simulink model "PreCNN_SAC_RL_env"  (R2025b)
settings: Solver=ode4  StartTime=0.0  StopTime=50  FixedStep=0.005  RelTol=1e-3  EnableMultiTasking=on
values from neighbouring files (symbols this model uses):
  dyn_obs = struct('p0', cell(1, num_dyn_obs), 'v', cell(1, num_dyn_obs), 'radius', cell(1, num_dyn_obs))    [genera_ostacoli_dinamici.m]    (also in visualizza_raggi_completo.m = scenario.dynamic_obstacles)
  initialGainsMultiplier = 15    [init_rl.m]    (also in report_agent.m; test.m; test_agent.m; train.m)
  logging = true    [train.m]    (also in train_agent.m; train_agent_precedente.m)
  Ts = 0.1    [init_rl.m]    (also in report_agent.m; test.m; test_agent.m; train.m)
undefined symbols (not defined in the file or in its folder): angControlTuning, angRateControlTuning, bounds, Controller, decyear, DiscIntNeverNeededParam, DroneMass, Dz, Gravity, initialConditions, Iz, leapyear, logPath_num, Nz, posControlTuning, Pz, startFlightTime, tunePositionController, UAVSampleTime, Vehicle, velControlTuning
libraries: slpidlib x14, slctrl_autotuning x8, sharedutil x4, aerolibconvert2 x3, aerolibatmos2 x2, aerolibgravity2 x2, shared6dof x2, aerolibasang x2, sensorinslib x2, deeplib x1, rllib x1, matrix_library x1
(part 3 of 5)

== system PreCNN_SAC_RL_env/Inner Loop and Plant Model/High-FidelityModel/Plant Model/Bus setup/Generate GPS Data ==
  XYZ (NEU) : Inport
  "Vx, Vy, Vz" : Inport  Port=2
  DCM : Inport  Port=3
  Data Type Conversion : DataTypeConversion  OutDataTypeStr=double  SaturateOnIntegerOverflow=off  RndMeth=Floor
  Data Type Conversion1 : DataTypeConversion  OutDataTypeStr=double  SaturateOnIntegerOverflow=off  RndMeth=Floor
  GPS Model : sensorinslib/INS  Commented=through  MountingLocation=[0 0 0]  RollAccuracy=0.2  PitchAccuracy=0.2  YawAccuracy=1  PositionAccuracy=0.85  VelocityAccuracy=0.05  UseAccelAndAngVel=off  AccelerationAccuracy=0  AngularVelocityAccuracy=0  TimeInput=off  PositionErrorFactor=[0 0 0]  SeedDouble=67  SimulateUsing=Code generation
  Reshape : Reshape  OutputDimensionality=Customize  OutputDimensions=[1 3]
  Reshape1 : Reshape  OutputDimensionality=Customize  OutputDimensions=[1 3]
  "Scale and Assemble GPS Data " : Subsystem
  Terminator1 : Terminator
  Variant Source : VariantSource  VariantControlMode=label  LabelModeActiveChoice=Model  VariantControls={NoModel, Model}
  Variant Source1 : VariantSource  VariantControlMode=label  LabelModeActiveChoice=Model  VariantControls={NoModel, Model}
  GPSData : Outport  VectorParamsAs1DForOutWhenUnconnected=off
  wires:
  DCM/1 -> GPS Model/3
  "Vx, Vy, Vz"/1 -> Variant Source1/1, Reshape1/1
  XYZ (NEU)/1 -> Variant Source/1, Reshape/1
  GPS Model/3 -> Terminator1/1
  Reshape/1 -> GPS Model/1
  Reshape1/1 -> GPS Model/2
  "Scale and Assemble GPS Data "/1(Out1) -> GPSData/1
  GPS Model/1 -> Data Type Conversion1/1
  Variant Source1/1 -> "Scale and Assemble GPS Data "/2(Ve)
  GPS Model/2 -> Data Type Conversion/1
  Variant Source/1 -> "Scale and Assemble GPS Data "/1(Xe)
  Data Type Conversion/1 -> Variant Source1/2
  Data Type Conversion1/1 -> Variant Source/2

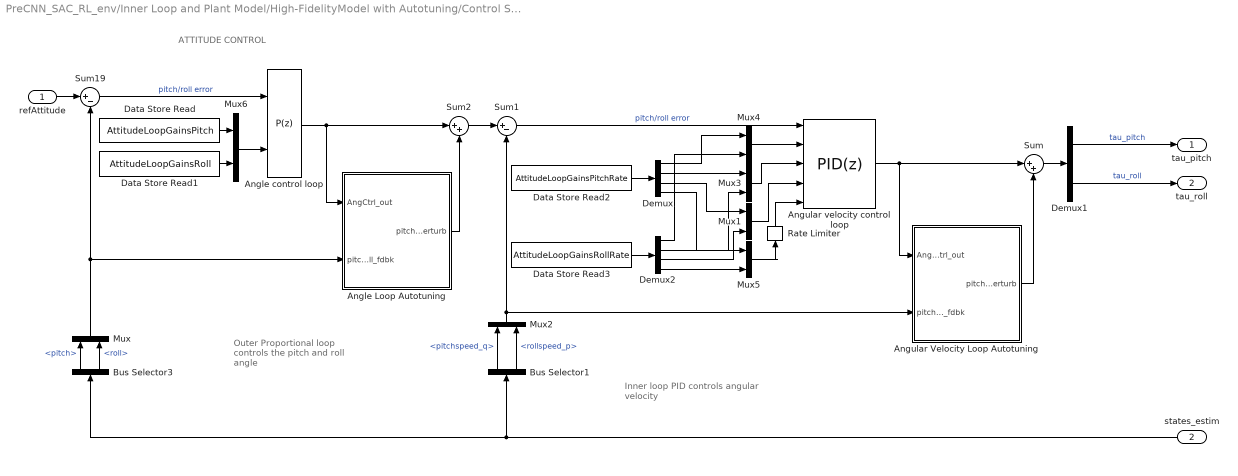
== system PreCNN_SAC_RL_env/Inner Loop and Plant Model/High-FidelityModel with Autotuning/Control System/Controller/Attitude Controller ==
  note: Inner loop PID
      | controls angular velocity
  note: Outer Proportional loop
      | controls the pitch and roll angle
  note: ATTITUDE CONTROL
  refAttitude : Inport
  states_estim : Inport  Port=2
  Angle Loop Autotuning : Subsystem
  Angle control loop : slpidlib/PID Controller  Controller=P  Form=Parallel  TimeDomain=Discrete-time  UseExternalTs=off  SampleTime=UAVSampleTime  IntegratorMethod=Forward Euler  FilterMethod=Forward Euler  ControllerParametersSource=external  P=5  I=1  UseKiTs=off  D=0  UseExternalDerivativeSource=off  N=100  UseFilter=on  TunerSelectOption=Transfer Function Based (PID Tuner App)  InitialConditionSource=internal  InitialConditionForIntegrator=0  InitialConditionForFilter=0  DifferentiatorICPrevScaledInput=0  ExternalReset=none  TrackingMode=off  Kt=1  LimitOutput=off  SatLimitsSource=internal  UpperSaturationLimit=inf  LowerSaturationLimit=-inf  LinearizeAsGain=on  AntiWindupMode=none  Kb=1  LimitIntegrator=off  UpperIntegratorSaturationLimit=inf  LowerIntegratorSaturationLimit=-inf  POutMin=[]  POutMax=[]  IOutMin=[]  IOutMax=[]  DOutMin=[]  DOutMax=[]  NOutMin=[]  NOutMax=[]  SumOutMin=[]  SumOutMax=[]  SaturationOutMin=[]  SaturationOutMax=[]  PParamMin=[]  PParamMax=[]  IParamMin=[]  IParamMax=[]  DParamMin=[]  DParamMax=[]  NParamMin=[]  NParamMax=[]  KbParamMin=[]  KbParamMax=[]  KtParamMin=[]  KtParamMax=[]  KbOutMin=[]  KbOutMax=[]  KtOutMin=[]  KtOutMax=[]  IntegratorOutMin=[]  IntegratorOutMax=[]  FilterOutMin=[]  FilterOutMax=[]  SumI1OutMin=[]  SumI1OutMax=[]  SumI2OutMin=[]  SumI2OutMax=[]  SumI3OutMin=[]  SumI3OutMax=[]  SumI4OutMin=[]  SumI4OutMax=[]  SumDOutMin=[]  SumDOutMax=[]  DifferentiatorOutMin=[]  DifferentiatorOutMax=[]  FilterDiffOutCoefMin=[]  FilterDiffOutCoefMax=[]  ReciprocalOutMin=[]  ReciprocalOutMax=[]  SumDenOutMin=[]  SumDenOutMax=[]  SumNumOutMin=[]  SumNumOutMax=[]  DivideOutMin=[]  DivideOutMax=[]  UdiffTsProdOutMin=[]  UdiffTsProdOutMax=[]  NTsProdOutMin=[]  NTsProdOutMax=[]  UintegralTsProdOutMin=[]  UintegralTsProdOutMax=[]  UngainTsProdOutMin=[]  UngainTsProdOutMax=[]  ClampingZeroOutDataTypeStr=Inherit: Inherit via back propagation  ClampingZeroOutMin=[]  ClampingZeroOutMax=[]  FilterDenConstantOutDataTypeStr=Inherit: Inherit via back propagation  FilterDenConstantOutMin=[]  FilterDenConstantOutMax=[]  PCopyOutDataTypeStr=Inherit: Inherit via back propagation  PCopyOutMin=[]  PCopyOutMax=[]  NCopyOutDataTypeStr=Inherit: Inherit via back propagation  NCopyOutMin=[]  NCopyOutMax=[]  IntegratorContinuousStateAttributes=''  IntegratorStateMustResolveToSignalObject=off  IntegratorRTWStateStorageClass=Auto  FilterContinuousStateAttributes=''  FilterStateMustResolveToSignalObject=off  FilterRTWStateStorageClass=Auto  ParallelPVariant=ExternalParameters  IdealPVariant=Disabled  IVariant=Disabled  DVariant=Disabled  IntegratorVariant=Disabled  SatVariant=Disabled  AWVariant=Disabled  PCopyVariant=Disabled  TRVariant=Disabled  FdbkBlocksVariant=Forward  IdealPFdbkVariant=Disabled  SatFdbkVariant=Disabled  DerivativeFilterVariant=Disabled  NVariant=Disabled  NCopyVariant=Disabled_SignalSpec  FilterICVariant=Disabled  IntegratorICVariant=Disabled  ExternalResetVariant=Disabled  TRSumVariant=Passthrough  SumFdbkVariant=Disabled  SumVariant=Passthrough_P  TsampFilterVariant=InternalTs  TsampNgainVariant=Passthrough  TsampIntegralVariant=Disabled_SignalSpec  ExternalSaturationOutDataTypeStr=Inherit: Same as second input  DerivativeSourceVariant=Disabled  PreIntVariant=InternalPreInt
  Angular Velocity Loop Autotuning : Subsystem
  Angular velocity control loop : slpidlib/PID Controller  Controller=PID  Form=Parallel  TimeDomain=Discrete-time  UseExternalTs=off  SampleTime=UAVSampleTime  IntegratorMethod=Forward Euler  FilterMethod=Forward Euler  ControllerParametersSource=external  P=[0.0025 .002]  I=[2*0.0025 0.003]  UseKiTs=off  D=[0.0025/25 0.003/50]  UseExternalDerivativeSource=off  N=70  UseFilter=on  TunerSelectOption=Transfer Function Based (PID Tuner App)  InitialConditionSource=internal  InitialConditionForIntegrator=0  InitialConditionForFilter=0  DifferentiatorICPrevScaledInput=0  ExternalReset=none  TrackingMode=off  Kt=1  LimitOutput=on  SatLimitsSource=internal  UpperSaturationLimit=20*pi/180  LowerSaturationLimit=-20*pi/180  LinearizeAsGain=on  AntiWindupMode=clamping  Kb=1  LimitIntegrator=off  UpperIntegratorSaturationLimit=inf  LowerIntegratorSaturationLimit=-inf  POutMin=[]  POutMax=[]  IOutMin=[]  IOutMax=[]  DOutMin=[]  DOutMax=[]  NOutMin=[]  NOutMax=[]  SumOutMin=[]  SumOutMax=[]  SaturationOutMin=[]  SaturationOutMax=[]  PParamMin=[]  PParamMax=[]  IParamMin=[]  IParamMax=[]  DParamMin=[]  DParamMax=[]  NParamMin=[]  NParamMax=[]  KbParamMin=[]  KbParamMax=[]  KtParamMin=[]  KtParamMax=[]  KbOutMin=[]  KbOutMax=[]  KtOutMin=[]  KtOutMax=[]  IntegratorOutMin=[]  IntegratorOutMax=[]  FilterOutMin=[]  FilterOutMax=[]  SumI1OutMin=[]  SumI1OutMax=[]  SumI2OutMin=[]  SumI2OutMax=[]  SumI3OutMin=[]  SumI3OutMax=[]  SumI4OutMin=[]  SumI4OutMax=[]  SumDOutMin=[]  SumDOutMax=[]  DifferentiatorOutMin=[]  DifferentiatorOutMax=[]  FilterDiffOutCoefMin=[]  FilterDiffOutCoefMax=[]  ReciprocalOutMin=[]  ReciprocalOutMax=[]  SumDenOutMin=[]  SumDenOutMax=[]  SumNumOutMin=[]  SumNumOutMax=[]  DivideOutMin=[]  DivideOutMax=[]  UdiffTsProdOutMin=[]  UdiffTsProdOutMax=[]  NTsProdOutMin=[]  NTsProdOutMax=[]  UintegralTsProdOutMin=[]  UintegralTsProdOutMax=[]  UngainTsProdOutMin=[]  UngainTsProdOutMax=[]  ClampingZeroOutDataTypeStr=Inherit: Inherit via back propagation  ClampingZeroOutMin=[]  ClampingZeroOutMax=[]  FilterDenConstantOutDataTypeStr=Inherit: Inherit via back propagation  FilterDenConstantOutMin=[]  FilterDenConstantOutMax=[]  PCopyOutDataTypeStr=Inherit: Inherit via back propagation  PCopyOutMin=[]  PCopyOutMax=[]  NCopyOutDataTypeStr=Inherit: Inherit via back propagation  NCopyOutMin=[]  NCopyOutMax=[]  IntegratorContinuousStateAttributes=''  IntegratorStateMustResolveToSignalObject=off  IntegratorRTWStateStorageClass=Auto  FilterContinuousStateAttributes=''  FilterStateMustResolveToSignalObject=off  FilterRTWStateStorageClass=Auto  ParallelPVariant=ExternalParameters  IdealPVariant=Disabled  IVariant=ExternalParameters  DVariant=ExternalParameters  IntegratorVariant=Discrete  SatVariant=Enabled  AWVariant=DiscClampingParallel  PCopyVariant=Disabled  TRVariant=Disabled  FdbkBlocksVariant=Forward  IdealPFdbkVariant=Disabled  SatFdbkVariant=Disabled  DerivativeFilterVariant=ForwardEulerFilter  NVariant=ExternalParameters  NCopyVariant=Disabled  FilterICVariant=InternalICsFilter  IntegratorICVariant=InternalICs  ExternalResetVariant=Disabled  TRSumVariant=Passthrough  SumFdbkVariant=Disabled  SumVariant=Sum_PID  TsampFilterVariant=InternalTs  TsampNgainVariant=Passthrough  TsampIntegralVariant=Disabled_SignalSpec  ExternalSaturationOutDataTypeStr=Inherit: Same as second input  DerivativeSourceVariant=ErrorSignal  PreIntVariant=InternalPreInt
  Bus Selector1 : BusSelector  OutputSignals=attitude.pitchspeed_q,attitude.rollspeed_p
  Bus Selector3 : BusSelector  OutputSignals=attitude.pitch,attitude.roll
  Data Store Read : DataStoreRead  DataStoreName=AttitudeLoopGainsPitch  IndexOptions=Index vector (dialog)  Indices=1  OutputSizes=1
  Data Store Read1 : DataStoreRead  DataStoreName=AttitudeLoopGainsRoll  IndexOptions=Index vector (dialog)  Indices=1  OutputSizes=1
  Data Store Read2 : DataStoreRead  DataStoreName=AttitudeLoopGainsPitchRate  IndexOptions=Index vector (dialog)  Indices=1  OutputSizes=1
  Data Store Read3 : DataStoreRead  DataStoreName=AttitudeLoopGainsRollRate  IndexOptions=Index vector (dialog)  Indices=1  OutputSizes=1
  Demux : Demux
  Demux1 : Demux  Outputs=2
  Demux2 : Demux
  Mux{,1..6} (7 alike) : Mux  Inputs=2
  Rate Limiter : RateLimiter  RisingSlewLimit=1000  FallingSlewLimit=-1000  SampleTimeMode=inherited
  Sum : Sum  Inputs=|++
  Sum1 : Sum  Inputs=|+-
  Sum19 : Sum  Inputs=|+-
  Sum2 : Sum  Inputs=|++
  tau_pitch : Outport  VectorParamsAs1DForOutWhenUnconnected=off
  tau_roll : Outport  Port=2  VectorParamsAs1DForOutWhenUnconnected=off
  wires:
  Sum1/1 -> Angular velocity control loop/1  "pitch/roll error"
  Mux2/1 -> Sum1/2, Angular Velocity Loop Autotuning/2(pitchrollrate_fdbk)
  Sum19/1 -> Angle control loop/1  "pitch/roll error"
  Demux1/2 -> tau_roll/1  "tau_roll"
  Demux1/1 -> tau_pitch/1  "tau_pitch"
  Bus Selector3/2 -> Mux/2  "<roll>"
  Mux/1 -> Angle Loop Autotuning/2(pitchroll_fdbk), Sum19/2
  states_estim/1 -> Bus Selector3/1, Bus Selector1/1
  Bus Selector3/1 -> Mux/1  "<pitch>"
  Bus Selector1/1 -> Mux2/1  "<pitchspeed_q>"
  Bus Selector1/2 -> Mux2/2  "<rollspeed_p>"
  Sum/1 -> Demux1/1
  Angular velocity control loop/1 -> Sum/1, Angular Velocity Loop Autotuning/1(AngVelCtrl_out)
  Angular Velocity Loop Autotuning/1(pitchrollrate_perturb) -> Sum/2
  Sum2/1 -> Sum1/1
  Angle Loop Autotuning/1(pitchroll_perturb) -> Sum2/2
  Angle control loop/1 -> Angle Loop Autotuning/1(AngCtrl_out), Sum2/1
  Data Store Read3/1 -> Demux2/1
  Data Store Read2/1 -> Demux/1
  Mux4/1 -> Angular velocity control loop/2
  Demux/1 -> Mux4/1
  Demux/2 -> Mux3/1
  Demux/3 -> Mux1/1
  Demux/4 -> Mux5/1
  Demux2/4 -> Mux5/2
  Demux2/3 -> Mux1/2
  Demux2/2 -> Mux3/2
  Demux2/1 -> Mux4/2
  Mux3/1 -> Angular velocity control loop/3
  Mux1/1 -> Angular velocity control loop/4
  Mux5/1 -> Rate Limiter/1
  refAttitude/1 -> Sum19/1
  Data Store Read1/1 -> Mux6/2
  Data Store Read/1 -> Mux6/1
  Mux6/1 -> Angle control loop/2
  Rate Limiter/1 -> Angular velocity control loop/5

== system PreCNN_SAC_RL_env/Inner Loop and Plant Model/High-FidelityModel with Autotuning/Control System/Controller/ControlMixer ==
  tau_pitch : Inport
  tau_roll : Inport  Port=2
  tau_yaw : Inport  Port=3
  totalThrust : Inport  Port=4
  Mux2 : Mux
  Product : Product  Multiplication=Matrix(*)  RndMeth=Zero
  TorqueTotalThrustToThrustPerMotor : Constant  Value=Controller.Q2Ts  OutDataTypeStr=single
  thrusts_refout : Outport  VectorParamsAs1DForOutWhenUnconnected=off
  wires:
  Product/1 -> thrusts_refout/1
  tau_roll/1 -> Mux2/4
  tau_yaw/1 -> Mux2/2
  totalThrust/1 -> Mux2/1
  TorqueTotalThrustToThrustPerMotor/1 -> Product/1
  Mux2/1 -> Product/2
  tau_pitch/1 -> Mux2/3

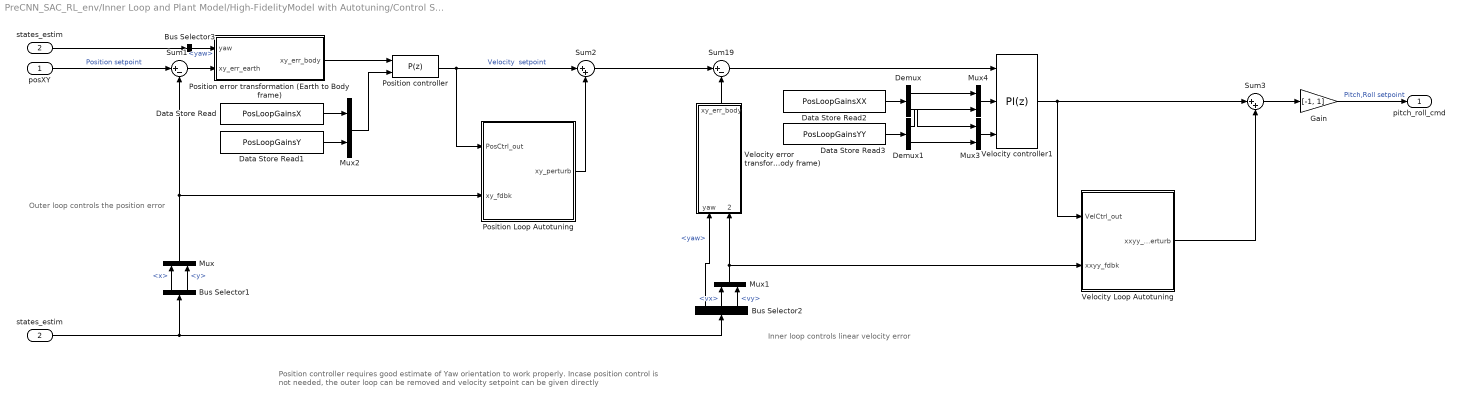
== system PreCNN_SAC_RL_env/Inner Loop and Plant Model/High-FidelityModel with Autotuning/Control System/Controller/Position Controller ==
  note: Outer loop controls the position error
  note: Inner loop controls linear velocity error
  note: Position controller requires good estimate of Yaw orientation to work properly.
      | Incase position control is not needed, the outer loop can be removed and velocity setpoint can be given directly
  posXY : Inport
  states_estim : Inport  Port=2
  Bus Selector1 : BusSelector  OutputSignals=pos_vel.x,pos_vel.y
  Bus Selector2 : BusSelector  OutputSignals=attitude.yaw,pos_vel.vx,pos_vel.vy
  Bus Selector3 : BusSelector  OutputSignals=attitude.yaw
  Data Store Read : DataStoreRead  DataStoreName=PosLoopGainsX  IndexOptions=Index vector (dialog)  Indices=1  OutputSizes=1
  Data Store Read1 : DataStoreRead  DataStoreName=PosLoopGainsY  IndexOptions=Index vector (dialog)  Indices=1  OutputSizes=1
  Data Store Read2 : DataStoreRead  DataStoreName=PosLoopGainsXX  IndexOptions=Index vector (dialog)  Indices=1  OutputSizes=1
  Data Store Read3 : DataStoreRead  DataStoreName=PosLoopGainsYY  IndexOptions=Index vector (dialog)  Indices=1  OutputSizes=1
  Demux : Demux  Outputs=2
  Demux1 : Demux  Outputs=2
  Gain : Gain  Gain=[-1, 1]
  Mux{,1..4} (5 alike) : Mux  Inputs=2
  Position Loop Autotuning : Subsystem
  Position controller : slpidlib/PID Controller  Controller=P  Form=Parallel  TimeDomain=Discrete-time  UseExternalTs=off  SampleTime=UAVSampleTime  IntegratorMethod=Forward Euler  FilterMethod=Forward Euler  ControllerParametersSource=external  P=0.25  I=0.1  UseKiTs=off  D=0  UseExternalDerivativeSource=off  N=100  UseFilter=on  TunerSelectOption=Transfer Function Based (PID Tuner App)  InitialConditionSource=internal  InitialConditionForIntegrator=0  InitialConditionForFilter=0  DifferentiatorICPrevScaledInput=0  ExternalReset=none  TrackingMode=off  Kt=1  LimitOutput=on  SatLimitsSource=internal  UpperSaturationLimit=4  LowerSaturationLimit=-4  LinearizeAsGain=on  AntiWindupMode=clamping  Kb=1  LimitIntegrator=off  UpperIntegratorSaturationLimit=inf  LowerIntegratorSaturationLimit=-inf  POutMin=[]  POutMax=[]  IOutMin=[]  IOutMax=[]  DOutMin=[]  DOutMax=[]  NOutMin=[]  NOutMax=[]  SumOutMin=[]  SumOutMax=[]  SaturationOutMin=[]  SaturationOutMax=[]  PParamMin=[]  PParamMax=[]  IParamMin=[]  IParamMax=[]  DParamMin=[]  DParamMax=[]  NParamMin=[]  NParamMax=[]  KbParamMin=[]  KbParamMax=[]  KtParamMin=[]  KtParamMax=[]  KbOutMin=[]  KbOutMax=[]  KtOutMin=[]  KtOutMax=[]  IntegratorOutMin=[]  IntegratorOutMax=[]  FilterOutMin=[]  FilterOutMax=[]  SumI1OutMin=[]  SumI1OutMax=[]  SumI2OutMin=[]  SumI2OutMax=[]  SumI3OutMin=[]  SumI3OutMax=[]  SumI4OutMin=[]  SumI4OutMax=[]  SumDOutMin=[]  SumDOutMax=[]  DifferentiatorOutMin=[]  DifferentiatorOutMax=[]  FilterDiffOutCoefMin=[]  FilterDiffOutCoefMax=[]  ReciprocalOutMin=[]  ReciprocalOutMax=[]  SumDenOutMin=[]  SumDenOutMax=[]  SumNumOutMin=[]  SumNumOutMax=[]  DivideOutMin=[]  DivideOutMax=[]  UdiffTsProdOutMin=[]  UdiffTsProdOutMax=[]  NTsProdOutMin=[]  NTsProdOutMax=[]  UintegralTsProdOutMin=[]  UintegralTsProdOutMax=[]  UngainTsProdOutMin=[]  UngainTsProdOutMax=[]  ClampingZeroOutDataTypeStr=Inherit: Inherit via back propagation  ClampingZeroOutMin=[]  ClampingZeroOutMax=[]  FilterDenConstantOutDataTypeStr=Inherit: Inherit via back propagation  FilterDenConstantOutMin=[]  FilterDenConstantOutMax=[]  PCopyOutDataTypeStr=Inherit: Inherit via back propagation  PCopyOutMin=[]  PCopyOutMax=[]  NCopyOutDataTypeStr=Inherit: Inherit via back propagation  NCopyOutMin=[]  NCopyOutMax=[]  IntegratorContinuousStateAttributes=''  IntegratorStateMustResolveToSignalObject=off  IntegratorRTWStateStorageClass=Auto  FilterContinuousStateAttributes=''  FilterStateMustResolveToSignalObject=off  FilterRTWStateStorageClass=Auto  ParallelPVariant=ExternalParameters  IdealPVariant=Disabled  IVariant=Disabled  DVariant=Disabled  IntegratorVariant=Disabled  SatVariant=Enabled  AWVariant=Disabled  PCopyVariant=Disabled  TRVariant=Disabled  FdbkBlocksVariant=Forward  IdealPFdbkVariant=Disabled  SatFdbkVariant=Disabled  DerivativeFilterVariant=Disabled  NVariant=Disabled  NCopyVariant=Disabled_SignalSpec  FilterICVariant=Disabled  IntegratorICVariant=Disabled  ExternalResetVariant=Disabled  TRSumVariant=Passthrough  SumFdbkVariant=Disabled  SumVariant=Passthrough_P  TsampFilterVariant=InternalTs  TsampNgainVariant=Passthrough  TsampIntegralVariant=Disabled_SignalSpec  ExternalSaturationOutDataTypeStr=Inherit: Same as second input  DerivativeSourceVariant=Disabled  PreIntVariant=InternalPreInt
  Position error transformation (Earth to Body frame) : MATLAB Function  TreatAsAtomicUnit=on
  Sum1 : Sum  Inputs=|+-
  Sum19 : Sum  Inputs=|+-
  Sum2 : Sum  Inputs=|++
  Sum3 : Sum  Inputs=|++
  Velocity Loop Autotuning : Subsystem
  Velocity controller1 : slpidlib/PID Controller  Controller=PI  Form=Parallel  TimeDomain=Discrete-time  UseExternalTs=off  SampleTime=UAVSampleTime  IntegratorMethod=Forward Euler  FilterMethod=Forward Euler  ControllerParametersSource=external  P=0.15  I=0.075  UseKiTs=off  D=0  UseExternalDerivativeSource=off  N=100  UseFilter=on  TunerSelectOption=Transfer Function Based (PID Tuner App)  InitialConditionSource=internal  InitialConditionForIntegrator=0  InitialConditionForFilter=0  DifferentiatorICPrevScaledInput=0  ExternalReset=none  TrackingMode=off  Kt=1  LimitOutput=on  SatLimitsSource=internal  UpperSaturationLimit=20*pi/180  LowerSaturationLimit=-20*pi/180  LinearizeAsGain=on  AntiWindupMode=clamping  Kb=1  LimitIntegrator=off  UpperIntegratorSaturationLimit=inf  LowerIntegratorSaturationLimit=-inf  POutMin=[]  POutMax=[]  IOutMin=[]  IOutMax=[]  DOutMin=[]  DOutMax=[]  NOutMin=[]  NOutMax=[]  SumOutMin=[]  SumOutMax=[]  SaturationOutMin=[]  SaturationOutMax=[]  PParamMin=[]  PParamMax=[]  IParamMin=[]  IParamMax=[]  DParamMin=[]  DParamMax=[]  NParamMin=[]  NParamMax=[]  KbParamMin=[]  KbParamMax=[]  KtParamMin=[]  KtParamMax=[]  KbOutMin=[]  KbOutMax=[]  KtOutMin=[]  KtOutMax=[]  IntegratorOutMin=[]  IntegratorOutMax=[]  FilterOutMin=[]  FilterOutMax=[]  SumI1OutMin=[]  SumI1OutMax=[]  SumI2OutMin=[]  SumI2OutMax=[]  SumI3OutMin=[]  SumI3OutMax=[]  SumI4OutMin=[]  SumI4OutMax=[]  SumDOutMin=[]  SumDOutMax=[]  DifferentiatorOutMin=[]  DifferentiatorOutMax=[]  FilterDiffOutCoefMin=[]  FilterDiffOutCoefMax=[]  ReciprocalOutMin=[]  ReciprocalOutMax=[]  SumDenOutMin=[]  SumDenOutMax=[]  SumNumOutMin=[]  SumNumOutMax=[]  DivideOutMin=[]  DivideOutMax=[]  UdiffTsProdOutMin=[]  UdiffTsProdOutMax=[]  NTsProdOutMin=[]  NTsProdOutMax=[]  UintegralTsProdOutMin=[]  UintegralTsProdOutMax=[]  UngainTsProdOutMin=[]  UngainTsProdOutMax=[]  ClampingZeroOutDataTypeStr=Inherit: Inherit via back propagation  ClampingZeroOutMin=[]  ClampingZeroOutMax=[]  FilterDenConstantOutDataTypeStr=Inherit: Inherit via back propagation  FilterDenConstantOutMin=[]  FilterDenConstantOutMax=[]  PCopyOutDataTypeStr=Inherit: Inherit via back propagation  PCopyOutMin=[]  PCopyOutMax=[]  NCopyOutDataTypeStr=Inherit: Inherit via back propagation  NCopyOutMin=[]  NCopyOutMax=[]  IntegratorContinuousStateAttributes=''  IntegratorStateMustResolveToSignalObject=off  IntegratorRTWStateStorageClass=Auto  FilterContinuousStateAttributes=''  FilterStateMustResolveToSignalObject=off  FilterRTWStateStorageClass=Auto  ParallelPVariant=ExternalParameters  IdealPVariant=Disabled  IVariant=ExternalParameters  DVariant=Disabled  IntegratorVariant=Discrete  SatVariant=Enabled  AWVariant=DiscClampingParallel  PCopyVariant=Disabled  TRVariant=Disabled  FdbkBlocksVariant=Forward  IdealPFdbkVariant=Disabled  SatFdbkVariant=Disabled  DerivativeFilterVariant=Disabled  NVariant=Disabled  NCopyVariant=Disabled_SignalSpec  FilterICVariant=Disabled  IntegratorICVariant=InternalICs  ExternalResetVariant=Disabled  TRSumVariant=Passthrough  SumFdbkVariant=Disabled  SumVariant=Sum_PI  TsampFilterVariant=InternalTs  TsampNgainVariant=Passthrough  TsampIntegralVariant=Disabled_SignalSpec  ExternalSaturationOutDataTypeStr=Inherit: Same as second input  DerivativeSourceVariant=Disabled  PreIntVariant=InternalPreInt
  Velocity error transformation (Earth to Body frame) : MATLAB Function  TreatAsAtomicUnit=on
  "states_estim " : InportShadow  Port=2
  pitch_roll_cmd : Outport  VectorParamsAs1DForOutWhenUnconnected=off
  wires:
  Mux1/1 -> Velocity error transformation (Earth to Body frame)/2(xy_err_earth), Velocity Loop Autotuning/2(xxyy_fdbk)
  Bus Selector3/1 -> Position error transformation (Earth to Body frame)/1(yaw)  "<yaw>"
  posXY/1 -> Sum1/1  "Position setpoint"
  Position error transformation (Earth to Body frame)/1(xy_err_body) -> Position controller/1
  Mux/1 -> Sum1/2, Position Loop Autotuning/2(xy_fdbk)
  Position controller/1 -> Position Loop Autotuning/1(PosCtrl_out), Sum2/1  "Velocity  setpoint"
  Velocity controller1/1 -> Velocity Loop Autotuning/1(VelCtrl_out), Sum3/1
  Gain/1 -> pitch_roll_cmd/1  "Pitch,Roll setpoint"
  Sum19/1 -> Velocity controller1/1
  Bus Selector2/3 -> Mux1/2  "<vy>"
  Bus Selector1/2 -> Mux/2  "<y>"
  Bus Selector1/1 -> Mux/1  "<x>"
  states_estim/1 -> Bus Selector2/1, Bus Selector1/1
  Bus Selector2/2 -> Mux1/1  "<vx>"
  Bus Selector2/1 -> Velocity error transformation (Earth to Body frame)/1(yaw)  "<yaw>"
  "states_estim "/1 -> Bus Selector3/1
  Velocity error transformation (Earth to Body frame)/1(xy_err_body) -> Sum19/2
  Sum2/1 -> Sum19/1
  Position Loop Autotuning/1(xy_perturb) -> Sum2/2
  Sum3/1 -> Gain/1
  Velocity Loop Autotuning/1(xxyy_perturb) -> Sum3/2
  Sum1/1 -> Position error transformation (Earth to Body frame)/2(xy_err_earth)
  Data Store Read/1 -> Mux2/1
  Data Store Read1/1 -> Mux2/2
  Mux2/1 -> Position controller/2
  Data Store Read2/1 -> Demux/1
  Mux4/1 -> Velocity controller1/2
  Mux3/1 -> Velocity controller1/3
  Demux/1 -> Mux4/1
  Demux/2 -> Mux3/1
  Data Store Read3/1 -> Demux1/1
  Demux1/1 -> Mux4/2
  Demux1/2 -> Mux3/2

== system PreCNN_SAC_RL_env/Inner Loop and Plant Model/High-FidelityModel with Autotuning/Control System/Controller/Yaw Controller ==
  note: Yaw estimation is done solely using the gyroscope and it may drift with time.
  yaw_ref : Inport
  states_estim : Inport  Port=2
  Bus Selector1 : BusSelector  OutputSignals=attitude.yawspeed_r
  Bus Selector5 : BusSelector  OutputSignals=attitude.yaw
  D_yaw : Gain  Gain=.0006
  Discrete-Time Integrator : DiscreteIntegrator  gainval=1  SampleTime=-1  LimitOutput=on  UpperSaturationLimit=0.25  LowerSaturationLimit=-0.25  ICPrevOutput=DiscIntNeverNeededParam  ICPrevScaledInput=DiscIntNeverNeededParam
  I_yaw : Gain  Gain=0.002  ParamDataTypeStr=single  OutDataTypeStr=single
  MATLAB Function : MATLAB Function  TreatAsAtomicUnit=on
  MATLAB Function1 : MATLAB Function  TreatAsAtomicUnit=on
  P_yaw : Gain  Gain=0.006  ParamDataTypeStr=single  OutDataTypeStr=single
  Sum1 : Sum  Inputs=|+-  OutDataTypeStr=single  AccumDataTypeStr=single  SaturateOnIntegerOverflow=on
  Sum2 : Sum  Inputs=++-
  tau_yaw : Outport  VectorParamsAs1DForOutWhenUnconnected=off
  wires:
  MATLAB Function1/1(y) -> P_yaw/1, I_yaw/1
  MATLAB Function/1(y) -> Sum1/1
  Discrete-Time Integrator/1 -> Sum2/2
  yaw_ref/1 -> MATLAB Function/1(u)
  Sum1/1 -> MATLAB Function1/1(u)
  D_yaw/1 -> Sum2/3
  P_yaw/1 -> Sum2/1
  Bus Selector1/1 -> D_yaw/1  "<yawspeed_r>"
  states_estim/1 -> Bus Selector5/1, Bus Selector1/1
  Bus Selector5/1 -> Sum1/2  "<yaw>"
  Sum2/1 -> tau_yaw/1
  I_yaw/1 -> Discrete-Time Integrator/1

== system PreCNN_SAC_RL_env/Inner Loop and Plant Model/High-FidelityModel with Autotuning/Control System/Controller/gravity feedforward//equilibrium thrust ==
  note: ALTITUDE
  states_estim : Inport
  PosZ : Inport  Port=2
  Bus Selector1 : BusSelector  OutputSignals=pos_vel.z,pos_vel.vz
  D_z1 : Gain  Gain=0.75  ParamDataTypeStr=single  OutDataTypeStr=single  SaturateOnIntegerOverflow=on
  Discrete-Time Integrator : DiscreteIntegrator  SampleTime=UAVSampleTime  LimitOutput=on  UpperSaturationLimit=2  LowerSaturationLimit=-2  ICPrevOutput=DiscIntNeverNeededParam  ICPrevScaledInput=DiscIntNeverNeededParam
  I_pr : Gain  Gain=0.075
  P_z1 : Gain  Gain=0.65  ParamDataTypeStr=single  OutDataTypeStr=single  SaturateOnIntegerOverflow=on
  SaturationThrust1 : Saturate  UpperLimit=4*Controller.totalThrustMaxRelative*Controller.motorsThrustPerMotorMax  LowerLimit=-4*Controller.totalThrustMaxRelative*Controller.motorsThrustPerMotorMax  OutDataTypeStr=single
  Sum1 : Sum  Inputs=++-  OutDataTypeStr=single  AccumDataTypeStr=single  SaturateOnIntegerOverflow=on
  Sum2 : Sum  Inputs=+-|  OutDataTypeStr=single  AccumDataTypeStr=single  SaturateOnIntegerOverflow=on
  Sum5 : Sum  Inputs=++|  OutDataTypeStr=single  AccumDataTypeStr=single  SaturateOnIntegerOverflow=on
  w1 : Constant  Value=-Gravity*Vehicle.Airframe.mass  OutDataTypeStr=single
  altitude_cmd : Outport  VectorParamsAs1DForOutWhenUnconnected=off
  wires:
  I_pr/1 -> Discrete-Time Integrator/1
  Sum5/1 -> SaturationThrust1/1
  Discrete-Time Integrator/1 -> Sum1/1
  D_z1/1 -> Sum1/3  "dz"
  Sum2/1 -> I_pr/1, P_z1/1  "pitch/roll error"
  Bus Selector1/2 -> D_z1/1  "<vz>"
  P_z1/1 -> Sum1/2
  states_estim/1 -> Bus Selector1/1
  Bus Selector1/1 -> Sum2/2  "<z>"
  PosZ/1 -> Sum2/1
  Sum1/1 -> Sum5/2
  SaturationThrust1/1 -> altitude_cmd/1
  w1/1 -> Sum5/1

== system PreCNN_SAC_RL_env/Inner Loop and Plant Model/High-FidelityModel with Autotuning/Control System/Controller/thrustsToMotorCommands ==
  thrusts_refin : Inport
  MotorDirections : Gain  Gain=[1 -1 1 -1]
  Saturation5 : Saturate  UpperLimit=Vehicle.Motor.maxLimit  LowerLimit=Vehicle.Motor.minLimit
  ThrustToMotorCommand : Gain  Gain=-Vehicle.Motor.thrustToMotorCommand
  motors_cmdout : Outport  VectorParamsAs1DForOutWhenUnconnected=off
  wires:
  Saturation5/1 -> MotorDirections/1
  MotorDirections/1 -> motors_cmdout/1
  ThrustToMotorCommand/1 -> Saturation5/1
  thrusts_refin/1 -> ThrustToMotorCommand/1

== system PreCNN_SAC_RL_env/Inner Loop and Plant Model/High-FidelityModel with Autotuning/Plant Model/AC model/Applied Force Calculation ==
  gravity force : Inport  Unit=N
  Aerodynamic Forces : Inport  Port=2  Unit=N
  Motor Forces : Inport  Port=3  Unit=N
  Add1 : Sum  Inputs=+++
  Signal Specification : SignalSpecification  Dimensions=3
  External Forces : Outport  Unit=N  VectorParamsAs1DForOutWhenUnconnected=off
  wires:
  Add1/1 -> Signal Specification/1
  Motor Forces/1 -> Add1/3  "Motor Thrust"
  Aerodynamic Forces/1 -> Add1/2
  gravity force/1 -> Add1/1
  Signal Specification/1 -> External Forces/1

== system PreCNN_SAC_RL_env/Inner Loop and Plant Model/High-FidelityModel with Autotuning/Plant Model/AC model/Drag Calculation ==
  Density : Inport  Unit=kg/m^3
  Vb : Inport  Port=2  Unit=m/second
  Drag Calc : Subsystem
  Gain3 : Gain  Gain=-1
  Product : Product  RndMeth=Zero
  Sign : Signum  ZeroCross=off
  Drag : Outport  Unit=N  VectorParamsAs1DForOutWhenUnconnected=off
  wires:
  Density/1 -> Drag Calc/1(Density)
  Sign/1 -> Gain3/1
  Drag Calc/1(drag) -> Product/1
  Gain3/1 -> Product/2
  Product/1 -> Drag/1  "xDrag"
  Vb/1 -> Sign/1, Drag Calc/2(vel)

== system PreCNN_SAC_RL_env/Inner Loop and Plant Model/High-FidelityModel with Autotuning/Plant Model/AC model/Gravity Force Calculation ==
  DCMbe : Inport
  gravity : Inport  Port=2  Unit=m/s^2
  Gain1 : Gain  Gain=Vehicle.Airframe.mass
  Product : Product  Multiplication=Matrix(*)
  gravity force : Outport  Unit=N  VectorParamsAs1DForOutWhenUnconnected=off
  wires:
  gravity/1 -> Gain1/1
  Gain1/1 -> Product/2  "gravity force NED"
  Product/1 -> gravity force/1
  DCMbe/1 -> Product/1

== system PreCNN_SAC_RL_env/Inner Loop and Plant Model/High-FidelityModel with Autotuning/Plant Model/AC model/Motor Forces and Torques ==
  Vb : Inport
  Density : Inport  Port=2
  pqr : Inport  Port=3
  Motor Commands : Inport  Port=4
  D1 : Constant  Value=[Vehicle.Airframe.xy -Vehicle.Airframe.xy Vehicle.Airframe.h]
  D2 : Constant  Value=[Vehicle.Airframe.xy Vehicle.Airframe.xy Vehicle.Airframe.h]
  D3 : Constant  Value=[-Vehicle.Airframe.xy Vehicle.Airframe.xy Vehicle.Airframe.h]
  D4 : Constant  Value=[-Vehicle.Airframe.xy -Vehicle.Airframe.xy Vehicle.Airframe.h]
  For Each Subsystem : Subsystem  TreatAsAtomicUnit=on
  MotorsToW : Subsystem
  Sum of Elements : Sum  Inputs=+  CollapseMode=Specified dimension  CollapseDim=2
  Sum of Elements1 : Sum  Inputs=+  CollapseMode=Specified dimension  CollapseDim=2
  Vector Concatenate : Concatenate  NumInputs=4  Mode=Multidimensional array  ConcatenateDimension=2
  Motor Forces : Outport  Unit=N  VectorParamsAs1DForOutWhenUnconnected=off
  Motor Torques : Outport  Port=2  Unit=N*m  VectorParamsAs1DForOutWhenUnconnected=off
  wires:
  D4/1 -> Vector Concatenate/4
  MotorsToW/1(omegas_datout) -> For Each Subsystem/4(w)
  Vector Concatenate/1 -> For Each Subsystem/5(D)
  For Each Subsystem/2(Moments) -> Sum of Elements1/1
  pqr/1 -> For Each Subsystem/3(Omega)
  Vb/1 -> For Each Subsystem/1(Vb)
  Motor Commands/1 -> MotorsToW/1(motors_datin)
  D1/1 -> Vector Concatenate/1
  D3/1 -> Vector Concatenate/3
  D2/1 -> Vector Concatenate/2
  Sum of Elements1/1 -> Motor Torques/1
  Density/1 -> For Each Subsystem/2(rho)
  Sum of Elements/1 -> Motor Forces/1
  For Each Subsystem/1(Forces) -> Sum of Elements/1

== system PreCNN_SAC_RL_env/Inner Loop and Plant Model/High-FidelityModel with Autotuning/Plant Model/Bus setup/Generate GPS Data ==
  XYZ (NEU) : Inport
  "Vx, Vy, Vz" : Inport  Port=2
  DCM : Inport  Port=3
  GPS Model : sensorinslib/INS  MountingLocation=[0 0 0]  RollAccuracy=0.2  PitchAccuracy=0.2  YawAccuracy=1  PositionAccuracy=0.85  VelocityAccuracy=0.05  UseAccelAndAngVel=off  AccelerationAccuracy=0  AngularVelocityAccuracy=0  TimeInput=off  PositionErrorFactor=[0 0 0]  SeedDouble=67  SimulateUsing=Code generation
  Reshape : Reshape  OutputDimensionality=Customize  OutputDimensions=[1 3]
  Reshape1 : Reshape  OutputDimensionality=Customize  OutputDimensions=[1 3]
  "Scale and Assemble GPS Data " : Subsystem
  Terminator1 : Terminator
  Variant Source : VariantSource  VariantControlMode=label  LabelModeActiveChoice=Model  VariantControls={NoModel, Model}
  Variant Source1 : VariantSource  VariantControlMode=label  LabelModeActiveChoice=Model  VariantControls={NoModel, Model}
  GPSData : Outport  VectorParamsAs1DForOutWhenUnconnected=off
  wires:
  DCM/1 -> GPS Model/3
  "Vx, Vy, Vz"/1 -> Variant Source1/1, Reshape1/1
  XYZ (NEU)/1 -> Variant Source/1, Reshape/1
  GPS Model/3 -> Terminator1/1
  Reshape/1 -> GPS Model/1
  Reshape1/1 -> GPS Model/2
  "Scale and Assemble GPS Data "/1(Out1) -> GPSData/1
  GPS Model/1 -> Variant Source/2
  Variant Source1/1 -> "Scale and Assemble GPS Data "/2(Ve)
  GPS Model/2 -> Variant Source1/2
  Variant Source/1 -> "Scale and Assemble GPS Data "/1(Xe)

== system PreCNN_SAC_RL_env/Inner Loop and Plant Model/High-FidelityModel/Plant Model/AC model/Drag Calculation/Drag Calc ==
  Density : Inport  Unit=kg/m^3
  vel : Inport  Port=2  Unit=m/s
  Dynamic Pressure : aerolibasang/Dynamic Pressure
  Gain : Gain  Gain=[.25 .25]
  Mux1 : Mux  Inputs=2
  Product : Product  Inputs=3  RndMeth=Zero
  diameter : Constant  Value=Vehicle.Airframe.diameter  SampleTime=0
  dragCoeff : Constant  Value=Vehicle.Airframe.Cdx  SampleTime=0
  drag : Outport  Unit=N  VectorParamsAs1DForOutWhenUnconnected=off
  wires:
  Product/1 -> drag/1
  dragCoeff/1 -> Product/3  "Cd"
  Dynamic Pressure/1 -> Product/1  "q"
  diameter/1 -> Gain/1, Mux1/2
  Mux1/1 -> Product/2  "S"
  Gain/1 -> Mux1/1
  vel/1 -> Dynamic Pressure/1
  Density/1 -> Dynamic Pressure/2

== system PreCNN_SAC_RL_env/Inner Loop and Plant Model/High-FidelityModel/Plant Model/AC model/Motor Forces and Torques/For Each Subsystem ==
  Vb : Inport  PortDimensions=3
  rho : Inport  Port=2  PortDimensions=1
  Omega : Inport  Port=3
  w : Inport  Port=4  Partition=on  PartitionDimension=2  PartitionWidth=1  PartitionOffset=0
  D : Inport  Port=5  Partition=on  PartitionDimension=2  PartitionWidth=1  PartitionOffset=0
  For Each : ForEach  DisableCoverage=on
  RotorDynamics : Subsystem  TreatAsAtomicUnit=on
      mask init:
      | aeroicon('aeroblk');
      settings: RTWFcnNameOpts=Use subsystem name  RTWFileNameOpts=Use function name
  Forces : Outport  ConcatenationDimension=2  VectorParamsAs1DForOutWhenUnconnected=off
  Moments : Outport  Port=2  ConcatenationDimension=2  VectorParamsAs1DForOutWhenUnconnected=off
  wires:
  RotorDynamics/1(Fxyz) -> Forces/1
  RotorDynamics/2(Mxyz) -> Moments/1
  Vb/1 -> RotorDynamics/1(Vb)
  Omega/1 -> RotorDynamics/2(pqr)
  rho/1 -> RotorDynamics/3(rho)
  D/1 -> RotorDynamics/5(Arm)
  w/1 -> RotorDynamics/4(w)

== system PreCNN_SAC_RL_env/Inner Loop and Plant Model/High-FidelityModel/Plant Model/AC model/Motor Forces and Torques/MotorsToW ==
  motors_datin : Inport
  Motordirections : Gain  Gain=[1 -1 1 -1]  ParamDataTypeStr=single  OutDataTypeStr=Inherit: Inherit via back propagation  SaturateOnIntegerOverflow=on
  Motordirections1 : Gain  Gain=[1 -1 1 -1]  ParamDataTypeStr=single  OutDataTypeStr=Inherit: Inherit via back propagation  SaturateOnIntegerOverflow=on
  Saturation5 : Saturate  UpperLimit=Vehicle.Motor.maxLimit  LowerLimit=Vehicle.Motor.minLimit  OutDataTypeStr=Inherit: Inherit via back propagation
  Signed Sqrt : Sqrt  Operator=signedSqrt  OutDataTypeStr=Inherit: Inherit via back propagation
  motorsToW2_Gain : Gain  Gain=Vehicle.Motor.commandToW2Gain  ParamDataTypeStr=single  OutDataTypeStr=Inherit: Inherit via back propagation  SaturateOnIntegerOverflow=on
  omegas_datout : Outport  VectorParamsAs1DForOutWhenUnconnected=off
  wires:
  motorsToW2_Gain/1 -> Signed Sqrt/1
  Motordirections/1 -> Saturation5/1
  Saturation5/1 -> Motordirections1/1
  Motordirections1/1 -> motorsToW2_Gain/1
  Signed Sqrt/1 -> omegas_datout/1
  motors_datin/1 -> Motordirections/1

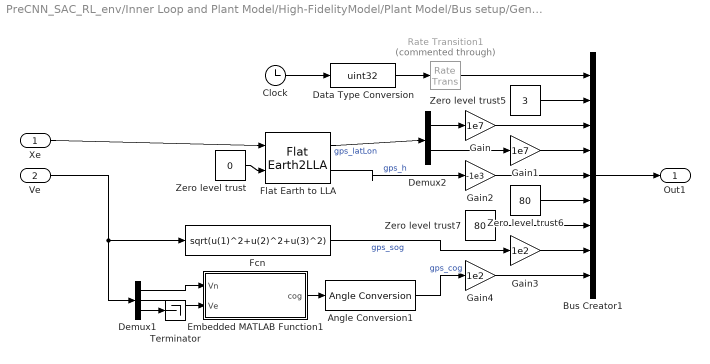
== system PreCNN_SAC_RL_env/Inner Loop and Plant Model/High-FidelityModel/Plant Model/Bus setup/Generate GPS Data/Scale and Assemble GPS Data  ==
  Xe : Inport
  Ve : Inport  Port=2
  Angle Conversion1 : aerolibconvert2/Angle Conversion  IU=rad  OU=deg
  Bus Creator1 : BusCreator  Inputs=9  OutDataTypeStr=Bus: gps_raw_int  NonVirtualBus=on
      settings: InheritFromInputs=off
  Clock : Clock
      settings: AttributesFormatString=Decimation: %<Decimation>
  Data Type Conversion : DataTypeConversion  OutDataTypeStr=uint32  SaturateOnIntegerOverflow=off  RndMeth=Floor
  Demux1 : Demux  Outputs=3
  Demux2 : Demux  Outputs=2
  Embedded MATLAB Function1 : MATLAB Function  TreatAsAtomicUnit=on
  Fcn : Fcn  Expr=sqrt(u(1)^2+u(2)^2+u(3)^2)
  Flat Earth to LLA : FlatEarth2LLA  R=6378137  LL0=uavIC_latLon
  Gain : Gain  Gain=1e7  OutDataTypeStr=int32
  Gain1 : Gain  Gain=1e7  OutDataTypeStr=int32
  Gain2 : Gain  Gain=-1e3  OutDataTypeStr=int32
  Gain3 : Gain  Gain=1e2  OutDataTypeStr=uint16
  Gain4 : Gain  Gain=1e2  OutDataTypeStr=uint16
  Rate Transition1 : RateTransition  Commented=through  OutPortSampleTime=0.005
  Terminator : Terminator
  Zero level trust : Constant  Value=0
      settings: AttributesFormatString=%<Value>
  Zero level trust5 : Constant  Value=3  OutDataTypeStr=uint8
      settings: AttributesFormatString=%<Value>
  Zero level trust6 : Constant  Value=80  OutDataTypeStr=uint16
      settings: AttributesFormatString=%<Value>
  Zero level trust7 : Constant  Value=80  OutDataTypeStr=uint16
      settings: AttributesFormatString=%<Value>
  Out1 : Outport
  wires:
  Demux2/1 -> Gain/1
  Gain/1 -> Bus Creator1/3
  Gain4/1 -> Bus Creator1/9
  Demux2/2 -> Gain1/1
  Embedded MATLAB Function1/1(cog) -> Angle Conversion1/1
  Rate Transition1/1 -> Bus Creator1/1
  Zero level trust6/1 -> Bus Creator1/6
  Gain3/1 -> Bus Creator1/8
  Clock/1 -> Data Type Conversion/1
  Ve/1 -> Demux1/1, Fcn/1
  Zero level trust7/1 -> Bus Creator1/7
  Data Type Conversion/1 -> Rate Transition1/1
  Demux1/2 -> Embedded MATLAB Function1/2(Ve)
  Zero level trust5/1 -> Bus Creator1/2
  Demux1/1 -> Embedded MATLAB Function1/1(Vn)
  Flat Earth to LLA/1 -> Demux2/1  "gps_latLon"
  Gain2/1 -> Bus Creator1/5
  Fcn/1 -> Gain3/1  "gps_sog"
  Gain1/1 -> Bus Creator1/4
  Flat Earth to LLA/2 -> Gain2/1  "gps_h"
  Zero level trust/1 -> Flat Earth to LLA/2
  Angle Conversion1/1 -> Gain4/1  "gps_cog"
  Demux1/3 -> Terminator/1
  Xe/1 -> Flat Earth to LLA/1
  Bus Creator1/1 -> Out1/1

== system PreCNN_SAC_RL_env/Inner Loop and Plant Model/High-FidelityModel with Autotuning/Control System/Controller/Attitude Controller/Angle Loop Autotuning ==
  AngCtrl_out : Inport
  pitchroll_fdbk : Inport  Port=2
  Closed-Loop PID Autotuner : slctrl_autotuning/Closed-Loop PID Autotuner  PIDType=P  PIDForm=Parallel  TimeDomain=discrete-time  DiscreteTs=UAVSampleTime  TuningTs=0.2  UseTuningTs=off  IntegratorFormula=Forward Euler  FilterFormula=Forward Euler  ContinuousTs=0.02  Bandwidth=angControlTuning.wc  UseExternalWC=off  TargetPM=angControlTuning.pm  UseExternalPM=off  UseExternalAchievedPM=off  ExperimentMode=Superposition  PlantType=Stable  PlantSign=Positive  AmpSine=angControlTuning.sineAmp  UseExternalAmpSine=off  UseExternalFRD=off  UseExternalU0=off  UseCompanion=off  NotDeployTuningModule=off  UsePLCCoder=off  OutputMode=perturbation only  BlockDataType=single  UseExperimentGoodPort=off  UseConnectedPID=on  blockpath=[]  tunedP=0  tunedI=0  tunedD=0  tunedN=100  tunedPM=0  EstimationWindowSize=3  UseExternalTuningParams=off  SingleMultiRateVariant=SingleSamplingRate  NumEstimationPeriods=4  NumSettlingPeriods=2  NumOfPRBSPeriod=1  PRBSSignalOrder=12  ExperimentModeVariant=VariantSuperimposed  OutputChoice=VariantDonly  ConvergenceCalcVariant=ConvSuperpositionPRBSVariant
  Closed-Loop PID Autotuner1 : slctrl_autotuning/Closed-Loop PID Autotuner  PIDType=P  PIDForm=Parallel  TimeDomain=discrete-time  DiscreteTs=UAVSampleTime  TuningTs=0.2  UseTuningTs=off  IntegratorFormula=Forward Euler  FilterFormula=Forward Euler  ContinuousTs=0.02  Bandwidth=angControlTuning.wc  UseExternalWC=off  TargetPM=angControlTuning.pm  UseExternalPM=off  UseExternalAchievedPM=off  ExperimentMode=Superposition  PlantType=Stable  PlantSign=Positive  AmpSine=angControlTuning.sineAmp  UseExternalAmpSine=off  UseExternalFRD=off  UseExternalU0=off  UseCompanion=off  NotDeployTuningModule=off  UsePLCCoder=off  OutputMode=perturbation only  BlockDataType=single  UseExperimentGoodPort=off  UseConnectedPID=on  blockpath=[]  tunedP=0  tunedI=0  tunedD=0  tunedN=100  tunedPM=0  EstimationWindowSize=3  UseExternalTuningParams=off  SingleMultiRateVariant=SingleSamplingRate  NumEstimationPeriods=4  NumSettlingPeriods=2  NumOfPRBSPeriod=1  PRBSSignalOrder=12  ExperimentModeVariant=VariantSuperimposed  OutputChoice=VariantDonly  ConvergenceCalcVariant=ConvSuperpositionPRBSVariant
  Display : Display
  Display1 : Display
  Mux : Mux  Inputs=2
  Scope : Scope
      settings: ActiveDisplayYMinimum=99.18257  ActiveDisplayYMaximum=100.62707  DataLoggingVariableName=ScopeData9
  Scope1 : Scope
      settings: DataLoggingVariableName=ScopeData10
  Selector : Selector  InputPortWidth=2  IndexOptions=Index vector (dialog)  Indices=1  OutputSizes=1
  Selector1 : Selector  InputPortWidth=2  IndexOptions=Index vector (dialog)  Indices=1  OutputSizes=1
  Selector2 : Selector  InputPortWidth=2  IndexOptions=Index vector (dialog)  Indices=2  OutputSizes=1
  Selector3 : Selector  InputPortWidth=2  IndexOptions=Index vector (dialog)  Indices=2  OutputSizes=1
  Step : Step  Time=angControlTuning.startExpRoll  SampleTime=UAVSampleTime
  Step1 : Step  Time=angControlTuning.stopExpRoll  After=-1  SampleTime=UAVSampleTime
  Step2 : Step  Time=angControlTuning.startExpPitch  SampleTime=UAVSampleTime
  Step3 : Step  Time=angControlTuning.stopExpPitch  After=-1  SampleTime=UAVSampleTime
  Sum : Sum  Inputs=|++
  Sum1 : Sum  Inputs=|++
  Update PID Gains : Subsystem
  pitchroll_perturb : Outport
  wires:
  Closed-Loop PID Autotuner1/3 -> Update PID Gains/4(PID Gains roll), Display1/1
  Closed-Loop PID Autotuner/3 -> Update PID Gains/1(PID Gains pitch), Display/1
  AngCtrl_out/1 -> Selector2/1, Selector/1
  pitchroll_fdbk/1 -> Selector3/1, Selector1/1
  Selector/1 -> Closed-Loop PID Autotuner/1
  Selector1/1 -> Closed-Loop PID Autotuner/2
  Sum/1 -> Update PID Gains/2(start/stop pitch), Closed-Loop PID Autotuner/3
  Step2/1 -> Sum/1
  Step3/1 -> Sum/2
  Closed-Loop PID Autotuner/2 -> Scope/1
  Mux/1 -> pitchroll_perturb/1
  Closed-Loop PID Autotuner/1 -> Mux/1
  Selector2/1 -> Closed-Loop PID Autotuner1/1
  Selector3/1 -> Closed-Loop PID Autotuner1/2
  Step1/1 -> Sum1/2
  Step/1 -> Sum1/1
  Sum1/1 -> Update PID Gains/3(start/stop roll), Closed-Loop PID Autotuner1/3
  Closed-Loop PID Autotuner1/2 -> Scope1/1
  Closed-Loop PID Autotuner1/1 -> Mux/2

== system PreCNN_SAC_RL_env/Inner Loop and Plant Model/High-FidelityModel with Autotuning/Control System/Controller/Attitude Controller/Angular Velocity Loop Autotuning ==
  AngVelCtrl_out : Inport
  pitchrollrate_fdbk : Inport  Port=2
  Closed-Loop PID Autotuner : slctrl_autotuning/Closed-Loop PID Autotuner  PIDType=PIDF  PIDForm=Parallel  TimeDomain=discrete-time  DiscreteTs=UAVSampleTime  TuningTs=0.2  UseTuningTs=off  IntegratorFormula=Forward Euler  FilterFormula=Forward Euler  ContinuousTs=0.02  Bandwidth=angRateControlTuning.wc  UseExternalWC=off  TargetPM=angRateControlTuning.pm  UseExternalPM=off  UseExternalAchievedPM=off  ExperimentMode=Superposition  PlantType=Stable  PlantSign=Positive  AmpSine=angRateControlTuning.sineAmp  UseExternalAmpSine=off  UseExternalFRD=off  UseExternalU0=off  UseCompanion=off  NotDeployTuningModule=off  UsePLCCoder=off  OutputMode=perturbation only  BlockDataType=single  UseExperimentGoodPort=off  UseConnectedPID=on  blockpath=[]  tunedP=0  tunedI=0  tunedD=0  tunedN=100  tunedPM=0  EstimationWindowSize=3  UseExternalTuningParams=off  SingleMultiRateVariant=SingleSamplingRate  NumEstimationPeriods=4  NumSettlingPeriods=2  NumOfPRBSPeriod=1  PRBSSignalOrder=12  ExperimentModeVariant=VariantSuperimposed  OutputChoice=VariantDonly  ConvergenceCalcVariant=ConvSuperpositionPRBSVariant
  Closed-Loop PID Autotuner1 : slctrl_autotuning/Closed-Loop PID Autotuner  PIDType=PIDF  PIDForm=Parallel  TimeDomain=discrete-time  DiscreteTs=UAVSampleTime  TuningTs=0.2  UseTuningTs=off  IntegratorFormula=Forward Euler  FilterFormula=Forward Euler  ContinuousTs=0.02  Bandwidth=angRateControlTuning.wc  UseExternalWC=off  TargetPM=angRateControlTuning.pm  UseExternalPM=off  UseExternalAchievedPM=off  ExperimentMode=Superposition  PlantType=Stable  PlantSign=Positive  AmpSine=angRateControlTuning.sineAmp  UseExternalAmpSine=off  UseExternalFRD=off  UseExternalU0=off  UseCompanion=off  NotDeployTuningModule=off  UsePLCCoder=off  OutputMode=perturbation only  BlockDataType=single  UseExperimentGoodPort=off  UseConnectedPID=on  blockpath=[]  tunedP=0  tunedI=0  tunedD=0  tunedN=100  tunedPM=0  EstimationWindowSize=3  UseExternalTuningParams=off  SingleMultiRateVariant=SingleSamplingRate  NumEstimationPeriods=4  NumSettlingPeriods=2  NumOfPRBSPeriod=1  PRBSSignalOrder=12  ExperimentModeVariant=VariantSuperimposed  OutputChoice=VariantDonly  ConvergenceCalcVariant=ConvSuperpositionPRBSVariant
  Display : Display
  Display1 : Display
  Mux : Mux  Inputs=2
  Scope : Scope
      settings: ActiveDisplayYMinimum=99.18257  ActiveDisplayYMaximum=100.62707  DataLoggingVariableName=ScopeData9
  Scope1 : Scope
      settings: DataLoggingVariableName=ScopeData10
  Selector : Selector  InputPortWidth=2  IndexOptions=Index vector (dialog)  Indices=1  OutputSizes=1
  Selector1 : Selector  InputPortWidth=2  IndexOptions=Index vector (dialog)  Indices=1  OutputSizes=1
  Selector2 : Selector  InputPortWidth=2  IndexOptions=Index vector (dialog)  Indices=2  OutputSizes=1
  Selector3 : Selector  InputPortWidth=2  IndexOptions=Index vector (dialog)  Indices=2  OutputSizes=1
  Step : Step  Time=angRateControlTuning.startExpRoll  SampleTime=UAVSampleTime
  Step1 : Step  Time=angRateControlTuning.stopExpRoll  After=-1  SampleTime=UAVSampleTime
  Step2 : Step  Time=angRateControlTuning.startExpPitch  SampleTime=UAVSampleTime
  Step3 : Step  Time=angRateControlTuning.stopExpPitch  After=-1  SampleTime=UAVSampleTime
  Sum : Sum  Inputs=|++
  Sum1 : Sum  Inputs=|++
  Update PID Gains : Subsystem
  pitchrollrate_perturb : Outport
  wires:
  Closed-Loop PID Autotuner1/1 -> Mux/2
  Closed-Loop PID Autotuner1/2 -> Scope1/1
  Sum1/1 -> Update PID Gains/3(start/stop rollrate), Closed-Loop PID Autotuner1/3
  Step/1 -> Sum1/1
  Step1/1 -> Sum1/2
  Selector3/1 -> Closed-Loop PID Autotuner1/2
  Selector2/1 -> Closed-Loop PID Autotuner1/1
  Closed-Loop PID Autotuner/1 -> Mux/1
  Mux/1 -> pitchrollrate_perturb/1
  Closed-Loop PID Autotuner/2 -> Scope/1
  Step3/1 -> Sum/2
  Step2/1 -> Sum/1
  Sum/1 -> Update PID Gains/2(start/stop pitchrate), Closed-Loop PID Autotuner/3
  Selector1/1 -> Closed-Loop PID Autotuner/2
  Selector/1 -> Closed-Loop PID Autotuner/1
  pitchrollrate_fdbk/1 -> Selector1/1, Selector3/1
  AngVelCtrl_out/1 -> Selector/1, Selector2/1
  Closed-Loop PID Autotuner/3 -> Update PID Gains/1(PID Gains pitchrate), Display/1
  Closed-Loop PID Autotuner1/3 -> Update PID Gains/4(PID Gains rollrate), Display1/1
